simulink model "systemDiagram"  (R2020a)
settings: Solver=VariableStepAuto  StartTime=0.0  StopTime=10.0  RelTol=1e-3
settings Model: Creator=robeshel  LastModifiedBy=Jiadoku

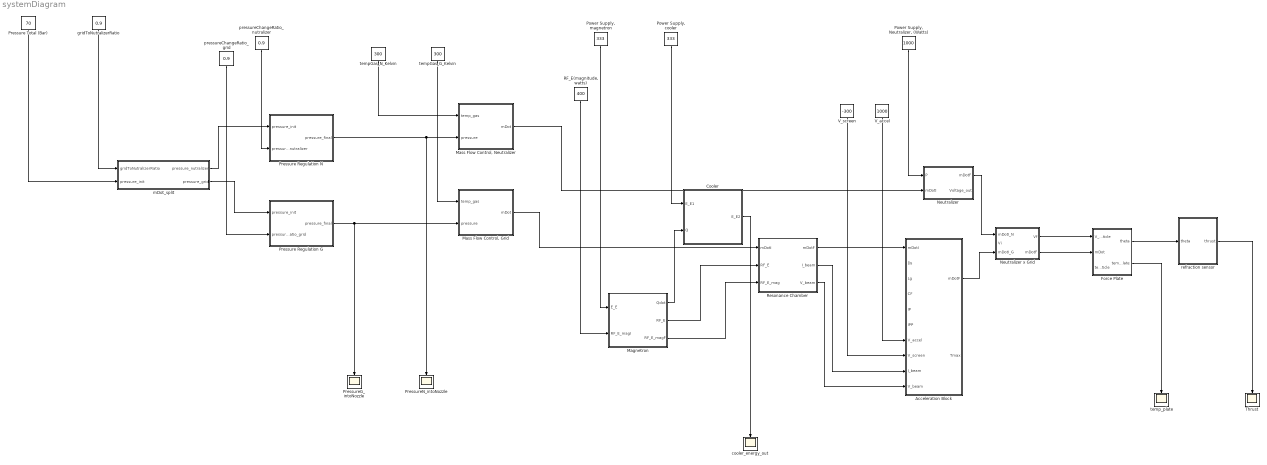
== system systemDiagram ==
  Acceleration Block : MATLAB Function  TreatAsAtomicUnit=on
  Cooler : MATLAB Function  TreatAsAtomicUnit=on
  Force Plate : MATLAB Function  TreatAsAtomicUnit=on
  Magnetron : MATLAB Function  TreatAsAtomicUnit=on
  "Mass Flow Control, Grid" : MATLAB Function  TreatAsAtomicUnit=on
  "Mass Flow Control, Neutralizer" : MATLAB Function  TreatAsAtomicUnit=on
  Neutralizer : MATLAB Function  TreatAsAtomicUnit=on
  Neutralizer x Grid : MATLAB Function  TreatAsAtomicUnit=on
  "Power Supply, Neutralizer, (Watts)" : Constant  Value=1000
  "Power Supply, cooler" : Constant  Value=333
  "Power Supply, magnetron" : Constant  Value=333
  Pressure Regulation G : MATLAB Function  TreatAsAtomicUnit=on
  Pressure Regulation N : MATLAB Function  TreatAsAtomicUnit=on
  Pressure Total (Bar) : Constant  Value=70
  PressureG_intoNozzle : Scope
  PressureN_intoNozzle : Scope
  "RF_E(magnitude, watts)" : Constant  Value=400
  Resonance Chamber : MATLAB Function  TreatAsAtomicUnit=on
  Thrust : Scope
  V_accel : Constant  Value=1000
  V_screen : Constant  Value=-300
  cooler_energy_out : Scope
  gridToNutralizerRatio : Constant  Value=0.9
  mDot_split : MATLAB Function  TreatAsAtomicUnit=on
  pressureChangeRatio_grid : Constant  Value=0.9
  pressureChangeRatio_nutralizer : Constant  Value=0.9
  refraction sensor : MATLAB Function  TreatAsAtomicUnit=on
  tempGas_G_Kelvin : Constant  Value=300
  tempGas_N_Kelvin : Constant  Value=300
  temp_plate : Scope
  wires:
  Neutralizer x Grid/1(Vf) -> Force Plate/1(V_particle)
  Neutralizer x Grid/2(mDotF) -> Force Plate/2(mDot)
  Neutralizer/1(mDotF) -> Neutralizer x Grid/1(mDotI_N)
  "Power Supply, Neutralizer, (Watts)"/1 -> Neutralizer/1(P)
  "Mass Flow Control, Neutralizer"/1(mDot) -> Neutralizer/2(mDotI)
  V_accel/1 -> Acceleration Block/7(V_accel)
  V_screen/1 -> Acceleration Block/8(V_screen)
  "Power Supply, magnetron"/1 -> Magnetron/1(E_E)
  Magnetron/1(Qdot) -> Cooler/2(Q)
  "Power Supply, cooler"/1 -> Cooler/1(E_E1)
  Acceleration Block/1(mDotF) -> Neutralizer x Grid/3(mDotI_G)
  refraction sensor/1(thrust) -> Thrust/1
  Force Plate/1(theta) -> refraction sensor/1(theta)
  Force Plate/2(temp_plate) -> temp_plate/1
  Cooler/1(E_E2) -> cooler_energy_out/1
  gridToNutralizerRatio/1 -> mDot_split/1(gridToNutralizerRatio)
  Pressure Total (Bar)/1 -> mDot_split/2(pressure_init)
  mDot_split/1(pressure_nutralizer) -> Pressure Regulation N/1("pressure_init ")
  mDot_split/2(pressure_grid) -> Pressure Regulation G/1(pressure_init)
  pressureChangeRatio_nutralizer/1 -> Pressure Regulation N/2(pressureChangeRatio_nutralizer)
  pressureChangeRatio_grid/1 -> Pressure Regulation G/2(pressureChangeRatio_grid)
  tempGas_N_Kelvin/1 -> "Mass Flow Control, Neutralizer"/1(temp_gas)
  tempGas_G_Kelvin/1 -> "Mass Flow Control, Grid"/1(temp_gas)
  Pressure Regulation N/1(pressure_final) -> PressureN_intoNozzle/1, "Mass Flow Control, Neutralizer"/2(pressure)
  Pressure Regulation G/1(pressure_final) -> "Mass Flow Control, Grid"/2(pressure), PressureG_intoNozzle/1
  "Mass Flow Control, Grid"/1(mDot) -> Resonance Chamber/1(mDotI)
  Resonance Chamber/1(mDotF) -> Acceleration Block/1(mDotI)
  Resonance Chamber/2(I_beam) -> Acceleration Block/9(I_beam)
  Resonance Chamber/3(V_beam) -> Acceleration Block/10(V_beam)
  Magnetron/2(RF_E) -> Resonance Chamber/2(RF_E)
  "RF_E(magnitude, watts)"/1 -> Magnetron/2(RF_E_magI)
  Magnetron/3(RF_E_magF) -> Resonance Chamber/3(RF_E_mag)

== matlab function systemDiagram/Pressure Regulation N ==
  data: pressure_init input; pressure_final output; pressureChangeRatio_nutralizer input
function pressure_final = fcn(pressure_init, pressureChangeRatio_nutralizer)

pressure_final = pressure_init * pressureChangeRatio_nutralizer;

== matlab function systemDiagram/Resonance Chamber ==
  data: mDotF output; I_beam output; mDotI input; RF_E input; RF_E_mag input; V_beam output
function [mDotF, I_beam, V_beam]= fcn(mDotI, RF_E, RF_E_mag)

%control--------------------------------------------------------------------------------
c=2.9*10^8;     %speed of light
f=2.45*10^9;%Hz of microwave
e=1.60218*10^-19;%charge of an electron
d_e=10^-18;%electron diameter
ep_0=1/(4*pi);%epsilon naught, vacuum permiativity
m=2.1801714*10^-25;%kg, mass of Xenon
k=1.38064852*10^-23; %m^2*kg*s^-2*K^-1 Boltzmann constant

%Independent--------------------------------------------------------------------------------
%magnetic field vector
Bv = ;

%initial charge density
L=sym('L');%length of chamber (most likely 5-10 cm)
Bv=sym('Bv');%magnetic field vector
%RF_E = sym('RF_E'); :: Electric field vector
phi=sym('phi');%reference potential

n_0=sym('n_0'); 
%phi=Q/(4*pi*ep_0*r^2)*exp(r/sqrt(ep_0*k*Te/(n_i*e^2))      %derived from
%n_0

% Q is total enclosed charge
z=54;%charge state and indenticle to A# as far as i can tell
v_e=sym('v_e');%electron velocity
Te=sym('Te');%Temperature of particle

%Dependent--------------------------------------------------------------------------------
%!!havn't gotten these yet!!
v_pa=sym('v_pa');%velocity parallel to the field
v_pe=sym('v_pe');%velocity perpandicular to the field
B=sym('B');%electric field strength, magnitude

n_e=n_0*exp(e*phi/k*Te);
charge_density=e*(z*n_i-n_e);
v_i=cross(RF_E,Bv)/B^2;%particle transverse velocity
%v=sqrt(v_pa^2+v_pe^2)
E_avg=1.5*k*Te;

Tev=Te*(e/k);%in ev instead of K
sigma_Xe=6.6*10^-19*(((Tev/4)-1)/(1+(Tev/4)^1.6));
%necassary equations
r_L=(1/B)*sqrt(2*m*v_pa/e);%radius of rotation around wavepath
t=v_pa/L;%%time to clear chamber (determined by mass flowrate)
x=sqrt(L^2+(2*pi*r_L*f*L/v_pe)^2);%total path length of particle

%needs to be optimized for a goal of 10% probability of collision
G_en=(n_e*sigma_Xe)^-1;
p=1-exp(-x/G_en);

%n = ;%degree of ionization of plasma
%t_e = ;%temperature of the electron
I_beam = (0.5* n) * ( e*sqrt( (k*t_e) / m) );%current density entering the sheath

mDotF = mDotI;

== matlab function systemDiagram/Magnetron ==
  data: E_E input; Qdot output; RF_E output; RF_E_magI input; RF_E_magF output
function [Qdot,RF_E, RF_E_magF]= fcn(E_E, RF_E_magI)

%X and R are number of iterations, increasing runtime

%IN------------------------------------------------------------------------
%electrical energy, power
Emanode=.2;%copper
Emchamber=.35;%ss
Sbcon=5.670373e-8; %W*m^-2*K^-4

%x is 1 second through 30 minutes
x=linspace(1,2100,2100);

%K

%temp of anode
T1= 1679.31+(-22252.17-1659.31)./(1+(x./1.881098e-39).^0.03126938);

%overall failure temp of anode
Tmax=150+273.15*ones(length(x));
hold on

%comparing heat to when it will fail
plot(x,T1)
plot(x,Tmax)

T2=298.15;
w=30*.0254;%"   %dimensions of chamber
h=50*.0254;%"

R=linspace(w,45*.0254,100);     %individual radia of points

%approximations of anode radius and length
%lanode=sym('Lanode');
lanode=.0508;
%ranode=sym('Ranode');
ranode=.0254;

%calculating temperature of each anode at the points from 1 second to 30 minutes
% and heat transfer from anode
for i=1:length(R)
for j=1:length(x)

A2=(pi*(w+h)/2)*lanode*3;   %area of chamber
A1=pi*ranode*lanode;        %area of anode

F(i,j)=A2./(pi.*R(i).^2);   %variable for radiative heat transfer

%taking into consideration emmisivity of the chamber and the anode (copper)
Den(i,j)=(1-Emanode)./(A1.*Emanode)+1./(A1.*F(i,j))+(1-Emchamber)./(A2.*Emchamber./2);

Qdot(i,j)=(Sbcon.*(T1(j).^4-T2.^4))./(Den(i,j));   %heat per second due to radiation

tREM(i,j)=T1(j)-Qdot(i,j);     %adjusted anode temperature
j=j+1;
end
i=i+1;
end

%can add work to conduction side of things

%OUT---------------------------------------------------------------------
%energy, creating microwaves that excite the xenon
%heat transfer (process inefficiencies)
T1= 1679.31+(-22252.17-1659.31)./(1+(x./1.881098e-39).^0.03126938);

RF_E = ;%electric field produced by the magnetron
RF_E_magF = RF_E_magI;

== matlab function systemDiagram/Cooler ==
  data: E_E1 input; E_E2 output; Q input
function E_E2 = fcn(E_E1, Q)


%IN---------------------------------------------------------------------
%Heat

%Power


%OUT---------------------------------------------------------------------
%Power (augmented)
%maybe has a -Q out, there will be a temperature difference between the
% cooler and the magnetron

== matlab function systemDiagram/mDot_split ==
  data: pressure_nutralizer output; pressure_grid output; gridToNutralizerRatio input; pressure_init input
function [pressure_nutralizer, pressure_grid]= fcn(gridToNutralizerRatio, pressure_init)

pressure_grid = pressure_init * gridToNutralizerRatio;
pressure_nutralizer = pressure_init * (1 - gridToNutralizerRatio);

== matlab function systemDiagram/Acceleration Block ==
  data: mDotF output; Tmax output; mDotI input; Ds input; Lg input; CF input; IP input; IPP input; V_accel input; V_screen input; I_beam input; V_beam input
function [mDotF, Tmax]= fcn(mDotI, Ds, Lg, CF, IP, IPP, V_accel, V_screen, I_beam, V_beam)

%Control variables-------------------------------------------------------------------------------
e = 1.60217662*(10^-19);                %charge of an electron
M = 2.1801714*(10^-25);                 %mass of a single xenon atom
epsilon = 8.8541878128*(10^-12);        %the permitivity of a vaccuum, farads/meter

%Independent variables------------------------------------------------------------
%Ds: diameter of screen grid holes

%Lg: distance between acceleration grid and screen grid.   !!Looking for optimal value!!

%!!NEED TO FIND!!
%CF: correction factor, correcting for the fact that the "ion current density" is not
% uniform.

%Ts: screen transparency                    !!NEED TO FIND!!

%!!POSSIBLE THE EQUATION MIKE IS LOOKING FOR!!
%I_beam: current of the ion beam            !!NEED TO FIND!!
%I_beam = (0.5* n) * ( e*sqrt( (k*t_e) / M) );


%V_beam: voltage of the ion beam            !!NEED TO FIND!!

%IP: current of the single charged ion;     !!NEED TO FIND!!

%IPP: current of the double charged ion;    !!NEED TO FIND!!

gamma = CF *( (Ip+1/sqrt(2)*Ipp)/(Ip+Ipp) );     %the corrected, average current of the ions

%Dependent variables-------------------------------------------------------------------------------
le = sqrt((Lg+Ts)^2+(Ds^2/4));  %distance between sheath and accelation grid

mDotF = mDotI;  %the rate of the mass passing through the grid must be 
                %equal to the rate of the mass entering the chamber

Vt = V_screen+abs(V_accel);      %V_screen is positive, V_accel is negative
Tmax = 4/9*(epsilon*gamma*Ts/e)*sqrt(2*e/M)*(Vt^(3/2)/le^2)*M*sqrt(2*e*Vb/M);

== matlab function systemDiagram/Neutralizer x Grid ==
  data: mDotI_N input; Vf output; mDotF output; Vi input; mDotI_G input
function [Vf,mDotF]= fcn(mDotI_N, Vi, mDotI_G)

Vf = Vi * 0.5;
if(mDotI_N > 100)
    mDotF = mDotI_G / 2;
end

== matlab function systemDiagram/Force Plate ==
  data: V_particle input; theta output; mDot input; temp_particle input; temp_plate output
function [theta, temp_plate] = fcn(V_particle, mDot, temp_particle)

%thrust equation of an ion engine
%theta = ;      !!NEED EQUATION!!


%Temperature of plate, Kelvin, xenon plasma is approx 6500K
%temp_plate = temp_particle * V_particle;     !!NEED EQUATION!!

== matlab function systemDiagram/Neutralizer ==
  data: P input; mDotI input; mDotF output; Voltage_out output
function [mDotF, Voltage_out] = fcn(P,mDotI)

mDotF = mDotI * P;

%Voltage_out = ;     !!NEED EQUATION!!

== matlab function systemDiagram/Mass Flow Control, Grid ==
  data: mDot output; temp_gas input; pressure input
function mDot = fcn(temp_gas, pressure)

%mDot = temp_gas * pressure;    !!NEED EQUATION!!

== matlab function systemDiagram/Mass Flow Control, Neutralizer ==
  data: mDot output; temp_gas input; pressure input
function mDot = fcn(temp_gas, pressure)

%mDot = temp_gas * pressure;    !!NEED EQUATION!!

== matlab function systemDiagram/Pressure Regulation G ==
  data: pressure_init input; pressure_final output; pressureChangeRatio_grid input
function pressure_final = fcn(pressure_init, pressureChangeRatio_grid)

pressure_final = pressure_init * pressureChangeRatio_grid;

== matlab function systemDiagram/refraction sensor ==
  data: theta input; thrust output
function thrust = fcn(theta)

%thrust = theta * ?;      !!NEED EQUATION!!
